simulink library "Hquad_control_LIB_MPC"  (Simulink 7.8)
settings: Solver=ode45  StartTime=0.0  StopTime=10.0  RelTol=1e-3
values from neighbouring files (symbols this model uses):
  FG_ctrl_x =     [kostas_malakies.mat]    (also in kostas_malakies2.mat)
  FG_ctrl_y =     [kostas_malakies.mat]    (also in kostas_malakies2.mat)
  FG_ctrl_yaw =     [kostas_malakies.mat]    (also in kostas_malakies2.mat)
  FG_ctrl_z =     [kostas_malakies.mat]    (also in kostas_malakies2.mat)
  g = 9.8065    [kostas_malakies.mat]    (also in kostas_malakies2.mat; load_PMModel.m = 9.81; main.m; main_last.m)
  kalm_mpc_x =     [kostas_malakies.mat]    (also in kostas_malakies2.mat)
  kalm_mpc_y =     [kostas_malakies.mat]    (also in kostas_malakies2.mat)
  kalm_mpc_yaw =     [kostas_malakies.mat]    (also in kostas_malakies2.mat)
  kalm_mpc_z =     [kostas_malakies.mat]    (also in kostas_malakies2.mat)
  MAX_BIAS_ANGLE = 0.0872664625997    [kostas_malakies.mat]    (also in kostas_malakies2.mat; main.m; main_last.m)
  MAX_BIAS_THRUST = 0.5    [kostas_malakies.mat]    (also in kostas_malakies2.mat; main.m; main_last.m)
  MAX_BIAS_YAW_RATE = 0.0872664625997    [kostas_malakies.mat]    (also in kostas_malakies2.mat; main.m; main_last.m)
  traj_FG =     [kostas.mat]    (also in kostas_malakies.mat; kostas_malakies2.mat; main_last.m = ReferenceCreator(maxdisty,maxdistz,scale_y,scale_z); traj_helix.mat)
  Ts = 0.02    [kostas_malakies.mat]    (also in kostas_malakies2.mat; main.m; main_last.m; matlab.mat = 0.08)
libraries: Hquad_control_LIB_MPC x17, simulink x9
(part 2 of 2)

== matlab function z controller MPC FG/runFastGradient ==
  data: TT_PP input double; u_opt output double; LL_PP input double; LL_ref_PP input double; LL_U_ref_PP input double; J_star output double; u_buff_out output double; V_init_out output double; MM input double; PP input double; AA_delay input double; BB_delay input double; x input double; X_ref input double; V_max input double; i_min input double; betas input double; L input double; u_buff input double; V_init input double
function [u_opt, J_star, u_buff_out, V_init_out] = fcn(TT_PP, LL_PP,...    
                        LL_ref_PP,LL_U_ref_PP, MM, PP, AA_delay, BB_delay, x, X_ref,...
                        V_max,i_min, betas, L, u_buff, V_init)

    % ugly, but simulink needs fix output sizes for vectors
    m = size(V_max,2); % number of outputs u
    delay_steps = size(BB_delay,2); % number of delay steps
    N = size(V_max,1); % prediction horizon
    
    % predict non-delayed state
    if(delay_steps==0)
        x_predicted=x;
    else
        x_predicted=AA_delay*x+BB_delay*u_buff;
    end
    
    % TODO get U_ref from trajectory
    U_ref=zeros(N,1);
    
    % set optimization variables
    LL_PP_ref=x_predicted'*LL_PP - X_ref'*LL_ref_PP - U_ref' * LL_U_ref_PP;
    MM_ref = x_predicted' * MM * x_predicted; % TODO expand to X_ref, U_ref
    
    % run fast gradient method
    [J_star, V_star, ~] = ...
        runFastGradient(TT_PP, LL_PP_ref, MM_ref, -V_max, V_max, V_init, ...
        i_min, betas, L, []);
    
    
    % Note: Fast gradient method is implemented in variable V where U = PP * V,
    % so don't forget to backtransform after termination:
    U_star = PP * V_star;

     % save outputs for delayed system
    if(delay_steps==0)
        u_buff_out=0;
    else
        u_buff_out=[u_buff(2:delay_steps,:); U_star(1:m,1)];
    end
 
    % set new initial guess
    V_init_out=[V_star(2:N);0];
    
    u_opt=U_star(1:m,1);

== matlab function yaw controller MPC FG/runFastGradient ==
  data: TT_PP input double; u_opt output double; LL_PP input double; LL_ref_PP input double; LL_U_ref_PP input double; J_star output double; u_buff_out output double; V_init_out output double; MM input double; PP input double; AA_delay input double; BB_delay input double; x input double; X_ref input double; V_max input double; i_min input double; betas input double; L input double; u_buff input double; V_init input double
function [u_opt, J_star, u_buff_out, V_init_out] = fcn(TT_PP, LL_PP,...    
                        LL_ref_PP,LL_U_ref_PP, MM, PP, AA_delay, BB_delay, x, X_ref,...
                        V_max,i_min, betas, L, u_buff, V_init)

    % ugly, but simulink needs fix output sizes for vectors
    m = size(V_max,2); % number of outputs u
    delay_steps = size(BB_delay,2); % number of delay steps
    N = size(V_max,1); % prediction horizon
    
    % predict non-delayed state
    if(delay_steps==0)
        x_predicted=x;
    else
        x_predicted=AA_delay*x+BB_delay*u_buff;
    end
    
    % TODO get U_ref from trajectory
    U_ref=zeros(N,1);
    
    % set optimization variables
    LL_PP_ref=x_predicted'*LL_PP - X_ref'*LL_ref_PP - U_ref' * LL_U_ref_PP;
    MM_ref = x_predicted' * MM * x_predicted; % TODO expand to X_ref, U_ref
    
    % run fast gradient method
    [J_star, V_star, ~] = ...
        runFastGradient(TT_PP, LL_PP_ref, MM_ref, -V_max, V_max, V_init, ...
        i_min, betas, L, []);
    
    
    % Note: Fast gradient method is implemented in variable V where U = PP * V,
    % so don't forget to backtransform after termination:
    U_star = PP * V_star;

     % save outputs for delayed system
    if(delay_steps==0)
        u_buff_out=0;
    else
        u_buff_out=[u_buff(2:delay_steps,:); U_star(1:m,1)];
    end
 
    % set new initial guess
    V_init_out=[V_star(2:N);0];
    
    u_opt=U_star(1:m,1);

== matlab function x states estimator bias/discrete kalman filter ==
  data: A input double; B input double; state_est output double; C input double; D input double; Q input double; R input double; u input double; y input double; P input double; state input double; P_est output double
function [state_est,P_est]  = fcn(A,B,C,D,Q,R, u, y, P, state)
%#eml

% Kalman filter according to Welch & Bishop, An Introduction to the Kalman
% Filter

n=size(A,1);

% Time update
x_=A*state+B*u;
P_=A*P*A'+Q;
  
% Measurement update
K=P_*C'*(C*P_*C'+R)^-1;
state_est=x_+K*(y-C*x_);
P_est=(eye(n)-K*C)*P_;

== matlab function z states estimator bias/discrete kalman filter ==
  data: A input double; B input double; state_est output double; C input double; D input double; Q input double; R input double; u input double; y input double; P input double; state input double; P_est output double
function [state_est,P_est]  = fcn(A,B,C,D,Q,R, u, y, P, state)
%#eml

% Kalman filter according to Welch & Bishop, An Introduction to the Kalman
% Filter

n=size(A,1);

% Time update
x_=A*state+B*u;
P_=A*P*A'+Q;
  
% Measurement update
K=P_*C'*(C*P_*C'+R)^-1;
state_est=x_+K*(y-C*x_);
P_est=(eye(n)-K*C)*P_;

== matlab function create ref traj from ref/generate_X_ref_x ==
  data: x_ref input double; x_dot_ref input double; X_ref output double
function X_ref  = fcn(x_ref, x_dot_ref)
   
pred_horizon=30;

X_ref_temp=[x_ref*ones(1,pred_horizon+1); x_dot_ref*ones(1,pred_horizon+1); zeros(1,pred_horizon+1)];

X_ref=reshape(X_ref_temp,1,[])';

== matlab function create ref traj from ref/generate_X_ref_y ==
  data: x_ref input double; x_dot_ref input double; X_ref output double
function X_ref  = fcn(x_ref, x_dot_ref)
   
pred_horizon=30;

X_ref_temp=[x_ref*ones(1,pred_horizon+1); x_dot_ref*ones(1,pred_horizon+1); zeros(1,pred_horizon+1)];

X_ref=reshape(X_ref_temp,1,[])';

== matlab function create ref traj from ref/generate_X_ref_yaw ==
  data: x_ref input double; x_dot_ref input double; X_ref output double
function X_ref  = fcn(x_ref, x_dot_ref)
   
pred_horizon=30;

X_ref_temp=[x_ref*ones(1,pred_horizon+1); x_dot_ref*ones(1,pred_horizon+1)];

X_ref=reshape(X_ref_temp,1,[])';

== matlab function create ref traj from ref/generate_X_ref_z ==
  data: x_ref input double; x_dot_ref input double; X_ref output double
function X_ref  = fcn(x_ref, x_dot_ref)
   
pred_horizon=30;

X_ref_temp=[x_ref*ones(1,pred_horizon+1); x_dot_ref*ones(1,pred_horizon+1)];

X_ref=reshape(X_ref_temp,1,[])';

== matlab function create ref traj/generate_X_ref_y ==
  data: traj_y input double; X_ref_y output double; idx input double
function X_ref_y  = fcn(traj_y,idx)

pred_horizon_y=30;

X_ref_y=traj_y(:,idx:idx+pred_horizon_y);

== matlab function create ref traj/generate_X_ref_yaw ==
  data: X_ref_yaw_unbounded input double; X_ref_yaw output double; yaw_meas input double; idx input double
function X_ref_yaw  = fcn(X_ref_yaw_unbounded,yaw_meas,idx)

pred_horizon_yaw=30;

yaw0=X_ref_yaw_unbounded(1,idx);
yaw_diff=yaw_meas-yaw0;


yaw_offset=round(yaw_diff/(2*pi))*2*pi;

X_ref_yaw=[X_ref_yaw_unbounded(1,idx:idx+pred_horizon_yaw)+yaw_offset;...
    X_ref_yaw_unbounded(2,idx:idx+pred_horizon_yaw)];

== matlab function create ref traj/generate_X_ref_z ==
  data: traj_z input double; X_ref_z output double; idx input double
function X_ref_z  = fcn(traj_z,idx)

pred_horizon_z=30;

X_ref_z=traj_z(:,idx:idx+pred_horizon_z);

== matlab function rotate to world frame/Embedded MATLAB Function ==
  data: roll input double; pitch input double; pitch_bias input double; roll_bias input double; roll_rot output double; yaw input double; pitch_rot output double; pitch_bias_rot output double; roll_bias_rot output double
function [roll_rot,pitch_rot,pitch_bias_rot,roll_bias_rot] = fcn(roll,pitch,pitch_bias,roll_bias,yaw)
%#eml


sin_yaw=sin(yaw);
cos_yaw=cos(yaw);

R=[cos_yaw, sin_yaw; -sin_yaw, cos_yaw];

temp=R*[pitch;roll];
pitch_rot=temp(1);
roll_rot=temp(2);

temp=R*[pitch_bias;roll_bias];
pitch_bias_rot=temp(1);
roll_bias_rot=temp(2);
